simulink model "MotorCC"  (R2019a)
settings: Solver=VariableStepAuto  StartTime=0.0  StopTime=35  RelTol=1e-3
libraries: vrlib x1
settings Model: Creator=julio  LastModifiedBy=julio

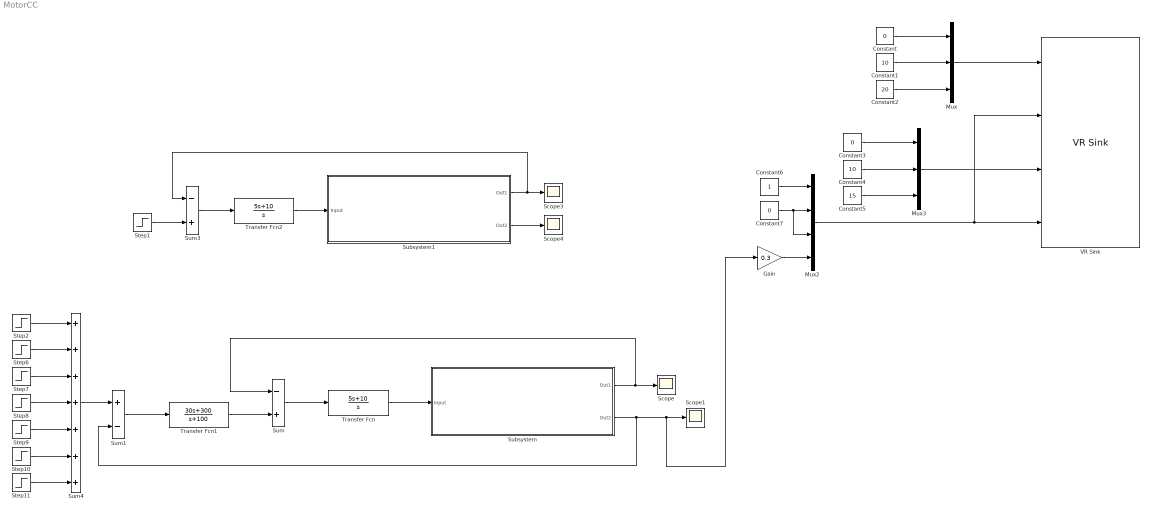
== system MotorCC ==
  Constant : Constant  Value=0
  Constant1 : Constant  Value=10
  Constant2 : Constant  Value=20
  Constant3 : Constant  Value=0
  Constant4 : Constant  Value=10
  Constant5 : Constant  Value=15
  Constant6 : Constant
  Constant7 : Constant  Value=0
  Gain : Gain  Gain=0.3
  Mux : Mux  Inputs=3
  Mux2 : Mux
  Mux3 : Mux  Inputs=3
  Scope{,1,3..4} (4 alike) : Scope
  Step1 : Step  SampleTime=0
  Step10 : Step  Time=25  Before=2  After=-2  SampleTime=5
  Step11 : Step  Time=30  Before=-2  After=0  SampleTime=5
  Step2 : Step  Time=0  After=3  SampleTime=5
  Step6 : Step  Time=5  Before=3  After=-3  SampleTime=5
  Step7 : Step  Time=10  Before=-3  After=1.5  SampleTime=5
  Step8 : Step  Time=15  Before=1.5  After=-1.5  SampleTime=5
  Step9 : Step  Time=20  Before=-1.5  After=2  SampleTime=5
  Subsystem : Subsystem  mask{kB=0.01, kM=0.02, kE=0.01, J=0.01, R=1, L=0.001}
      mask prompts: kB "Atrito viscoso"; kM "Cte mecanica"; kE "Cte eletrica"; J "Momento de inercia"; R "Resistencia eletrica"; L "Indutancia"
  Subsystem1 : Subsystem  mask{kB=0.01, kM=2, kE=1, J=1, R=10, L=0.1}
      mask prompts: kB "Atrito viscoso"; kM "Cte mecanica"; kE "Cte eletrica"; J "Momento de inercia"; R "Resistencia eletrica"; L "Indutancia"
  Sum : Sum  Inputs=-+
  Sum1 : Sum  Inputs=+-
  Sum3 : Sum  Inputs=-+
  Sum4 : Sum  Inputs=+++++++
  Transfer Fcn : TransferFcn  Numerator=[5 10]  Denominator=[1 0]
  Transfer Fcn1 : TransferFcn  Numerator=[30 300]  Denominator=[1 100]
  Transfer Fcn2 : TransferFcn  Numerator=[5 10]  Denominator=[1 0]
  VR Sink : vrlib/VR Sink  InstantiateOnLoad=on  SampleTime=0.1  ViewEnable=on  RemoteChange=off  RemoteView=off  FieldsWritten=Garra.center.3.1.1.double#Garra.rotation.4.1.1.double#Pincas.center.3.1.1.double#Pincas.rotation.4.1.1.double  WorldFileName=robotarm.wrl  AutoView=off  VideoDimensions=[]  AllowVariableSize=off
      settings: SourceProductName=Simulink
  wires:
  Transfer Fcn/1 -> Subsystem/1(Input)
  Sum/1 -> Transfer Fcn/1
  Subsystem/1(Out1) -> Sum/1, Scope/1
  Subsystem/2(Out2) -> Gain/1, Scope1/1, Sum1/2
  Transfer Fcn1/1 -> Sum/2
  Sum1/1 -> Transfer Fcn1/1
  Subsystem1/1(Out1) -> Sum3/1, Scope3/1
  Transfer Fcn2/1 -> Subsystem1/1(Input)
  Sum3/1 -> Transfer Fcn2/1
  Step1/1 -> Sum3/2
  Subsystem1/2(Out2) -> Scope4/1
  Constant1/1 -> Mux/2
  Constant/1 -> Mux/1
  Constant2/1 -> Mux/3
  Constant3/1 -> Mux3/1
  Constant4/1 -> Mux3/2
  Constant5/1 -> Mux3/3
  Mux/1 -> VR Sink/1
  Mux3/1 -> VR Sink/3
  Constant6/1 -> Mux2/1
  Constant7/1 -> Mux2/3, Mux2/2
  Gain/1 -> Mux2/4
  Mux2/1 -> VR Sink/2, VR Sink/4
  Step6/1 -> Sum4/2
  Step7/1 -> Sum4/3
  Step2/1 -> Sum4/1
  Step11/1 -> Sum4/7
  Step10/1 -> Sum4/6
  Step9/1 -> Sum4/5
  Step8/1 -> Sum4/4
  Sum4/1 -> Sum1/1

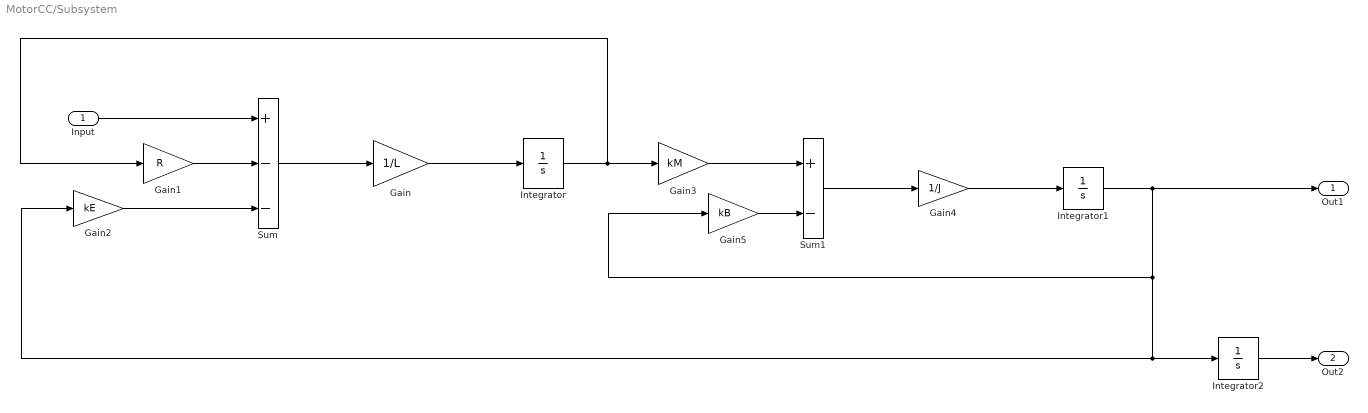
== system MotorCC/Subsystem ==
  Input : Inport
  Gain : Gain  Gain=1/L
  Gain1 : Gain  Gain=R
  Gain2 : Gain  Gain=kE
  Gain3 : Gain  Gain=kM
  Gain4 : Gain  Gain=1/J
  Gain5 : Gain  Gain=kB
  Integrator : Integrator
  Integrator1 : Integrator
  Integrator2 : Integrator
  Sum : Sum  Inputs=+--
  Sum1 : Sum  Inputs=+-
  Out1 : Outport
  Out2 : Outport  Port=2
  wires:
  Integrator1/1 -> Gain2/1, Integrator2/1, Gain5/1, Out1/1
  Integrator/1 -> Gain3/1, Gain1/1
  Gain/1 -> Integrator/1
  Gain1/1 -> Sum/2
  Sum1/1 -> Gain4/1
  Input/1 -> Sum/1
  Integrator2/1 -> Out2/1
  Gain4/1 -> Integrator1/1
  Sum/1 -> Gain/1
  Gain2/1 -> Sum/3
  Gain3/1 -> Sum1/1
  Gain5/1 -> Sum1/2

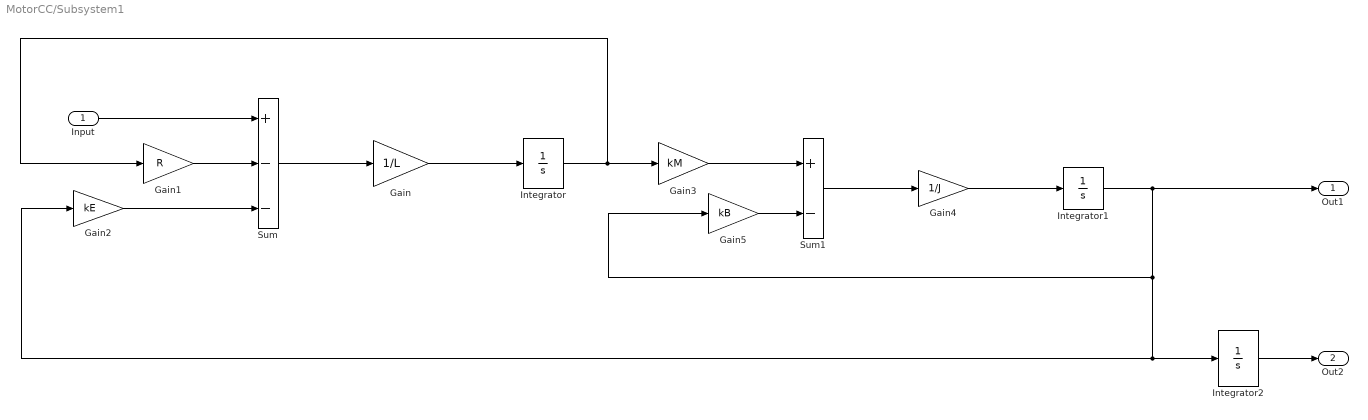
== system MotorCC/Subsystem1 ==
  Input : Inport
  Gain : Gain  Gain=1/L
  Gain1 : Gain  Gain=R
  Gain2 : Gain  Gain=kE
  Gain3 : Gain  Gain=kM
  Gain4 : Gain  Gain=1/J
  Gain5 : Gain  Gain=kB
  Integrator : Integrator
  Integrator1 : Integrator
  Integrator2 : Integrator
  Sum : Sum  Inputs=+--
  Sum1 : Sum  Inputs=+-
  Out1 : Outport
  Out2 : Outport  Port=2
  wires:
  Integrator1/1 -> Gain2/1, Integrator2/1, Gain5/1, Out1/1
  Integrator/1 -> Gain3/1, Gain1/1
  Gain/1 -> Integrator/1
  Gain1/1 -> Sum/2
  Sum1/1 -> Gain4/1
  Input/1 -> Sum/1
  Integrator2/1 -> Out2/1
  Gain4/1 -> Integrator1/1
  Sum/1 -> Gain/1
  Gain2/1 -> Sum/3
  Gain3/1 -> Sum1/1
  Gain5/1 -> Sum1/2
